simulink model "s_estudio_final"  (R2022b)
settings: Solver=VariableStepAuto  StartTime=0.0  StopTime=160.0  RelTol=1e-3
libraries: fuzblock x8, simulink x1
settings Model: Creator=sophy  LastModifiedBy=sophy

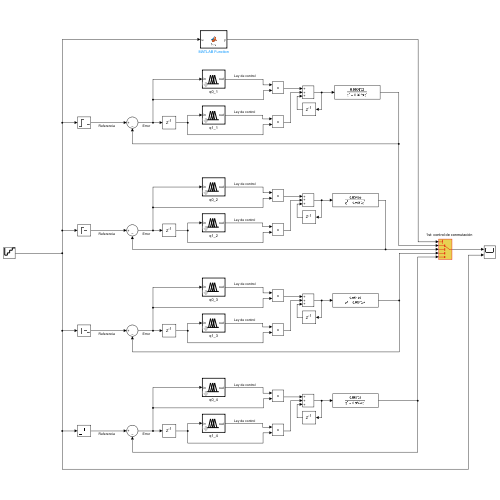
[thumbnail: Simulink's stored preview of the top-level diagram]
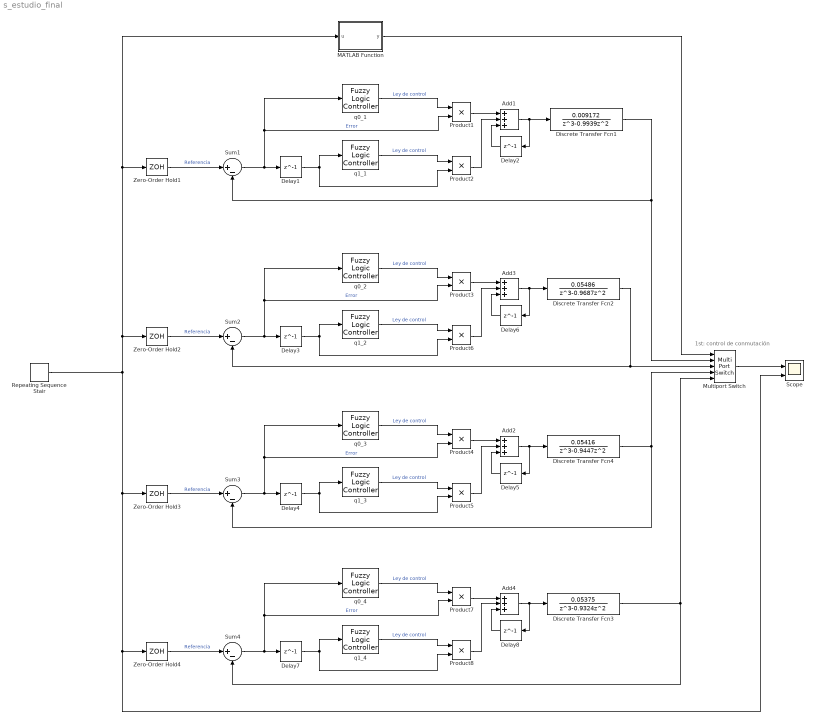
== system s_estudio_final ==
  note: 1st: control de conmutación
  Add{1..4} (4 alike) : Sum  Inputs=+++
  Delay{1..8} (8 alike) : Delay  DelayLength=1
  Discrete Transfer Fcn1 : DiscreteTransferFcn  Numerator=[0.009172]  Denominator=[1 -0.9939 0 0]
  Discrete Transfer Fcn2 : DiscreteTransferFcn  Numerator=[0.05486]  Denominator=[1 -0.9687 0 0]
  Discrete Transfer Fcn3 : DiscreteTransferFcn  Numerator=[0.05375]  Denominator=[1 -0.9324 0 0]
  Discrete Transfer Fcn4 : DiscreteTransferFcn  Numerator=[0.05416]  Denominator=[1 -0.9447 0 0]
  MATLAB Function : MATLAB Function  TreatAsAtomicUnit=on
  Multiport Switch : MultiPortSwitch  Inputs=4  SaturateOnIntegerOverflow=off  InputSameDT=off
  Product{1..8} (8 alike) : Product
  Repeating Sequence Stair : simulink/Sources/Repeating Sequence Stair  OutValues=[20 30 40 50].'  tsamp=40  OutMin=[]  OutMax=[]  OutDataTypeStr=double  OutputDataTypeScalingMode=double  OutDataType=fixdt(0,8)  ConRadixGroup=Best Precision: Vector-wise  OutScaling=2^-12
  Scope : Scope  NumInputPorts=2
  Sum{1..4} (4 alike) : Sum  Inputs=|+-
  Zero-Order Hold1 : ZeroOrderHold  SampleTime=0.2
  Zero-Order Hold2 : ZeroOrderHold  SampleTime=1.5303
  Zero-Order Hold3 : ZeroOrderHold  SampleTime=2.5897
  Zero-Order Hold4 : ZeroOrderHold  SampleTime=3.5
  q0_{1..4} (4 alike) : fuzblock/Fuzzy Logic  Controller  FIS=q0_PID  OutputSampleNumber=101  DataType=double  FuzzifiedInputs=off  RuleFiringStrengths=off  RuleOutputs=off  AggregatedOutputs=off  SimulateUsing=Interpreted execution  OutOfRangeInputValueMessage=warning  NoRuleFiredMessage=warning  EmptyOutputFuzzySetMessage=warning
  q1_{1..4} (4 alike) : fuzblock/Fuzzy Logic  Controller  FIS=q1_PID  OutputSampleNumber=101  DataType=double  FuzzifiedInputs=off  RuleFiringStrengths=off  RuleOutputs=off  AggregatedOutputs=off  SimulateUsing=Interpreted execution  OutOfRangeInputValueMessage=warning  NoRuleFiredMessage=warning  EmptyOutputFuzzySetMessage=warning
  wires:
  Product2/1 -> Add1/2
  Sum1/1 -> q0_1/1, Product1/2, Delay1/1  "Error"
  q0_1/1 -> Product1/1  "Ley de control"
  Zero-Order Hold1/1 -> Sum1/1  "Referencia"
  q1_1/1 -> Product2/1  "Ley de control"
  Add1/1 -> Delay2/1, Discrete Transfer Fcn1/1
  Delay7/1 -> Product8/2, q1_4/1
  Zero-Order Hold4/1 -> Sum4/1  "Referencia"
  Discrete Transfer Fcn4/1 -> Sum3/2, Multiport Switch/4
  Add2/1 -> Discrete Transfer Fcn4/1, Delay5/1
  Sum4/1 -> q0_4/1, Product7/2, Delay7/1  "Error"
  Product8/1 -> Add4/2
  Delay4/1 -> Product5/2, q1_3/1
  q1_3/1 -> Product5/1  "Ley de control"
  q0_4/1 -> Product7/1  "Ley de control"
  q0_3/1 -> Product4/1  "Ley de control"
  Delay5/1 -> Add2/3
  Discrete Transfer Fcn1/1 -> Sum1/2, Multiport Switch/2
  Add3/1 -> Delay6/1, Discrete Transfer Fcn2/1
  Zero-Order Hold3/1 -> Sum3/1  "Referencia"
  q1_2/1 -> Product6/1  "Ley de control"
  MATLAB Function/1(y) -> Multiport Switch/1
  Discrete Transfer Fcn3/1 -> Sum4/2, Multiport Switch/5
  Product4/1 -> Add2/1
  Delay8/1 -> Add4/3
  q0_2/1 -> Product3/1  "Ley de control"
  Zero-Order Hold2/1 -> Sum2/1  "Referencia"
  Discrete Transfer Fcn2/1 -> Sum2/2, Multiport Switch/3
  Product3/1 -> Add3/1
  Product7/1 -> Add4/1
  Delay6/1 -> Add3/3
  Product1/1 -> Add1/1
  Delay2/1 -> Add1/3
  Product5/1 -> Add2/2
  q1_4/1 -> Product8/1  "Ley de control"
  Product6/1 -> Add3/2
  Delay1/1 -> Product2/2, q1_1/1
  Sum2/1 -> q0_2/1, Product3/2, Delay3/1  "Error"
  Add4/1 -> Delay8/1, Discrete Transfer Fcn3/1
  Multiport Switch/1 -> Scope/1
  Delay3/1 -> Product6/2, q1_2/1
  Sum3/1 -> q0_3/1, Product4/2, Delay4/1  "Error"
  Repeating Sequence Stair/1 -> Zero-Order Hold1/1, MATLAB Function/1(u), Zero-Order Hold2/1, Zero-Order Hold3/1, Zero-Order Hold4/1, Scope/2

== matlab function s_estudio_final/MATLAB Function ==
  data: u input; y output
function y = fcn(u)

if ((u>0)&&(u<=20)) % u = lo que entra = escalon
u = 1; % activar pin 1
end

if ((u>20)&&(u<=30))
u = 2; % activar pin 2
end 

if ((u>30)&&(u<=40))
u = 3; % activar pin 3
end 

if ((u>40)&&(u<=50))
u = 4; % activar pin 4
end 

y = u;
